simulink model "discret"  (R2020a)
settings: Solver=VariableStepAuto  StartTime=0.0  StopTime=0.03  RelTol=1e-3
undefined symbols (not defined in the file): K, Kfiltre, S, Te, Tg, Tr1, Tr2, Ubatt, Z0, Z00, Z1, Z11
settings Model: Creator=housni  LastModifiedBy=housni

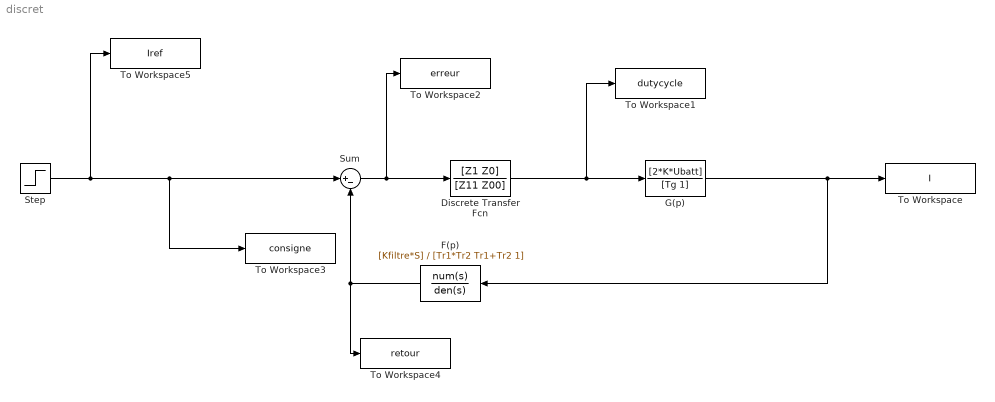
== system discret ==
  Discrete Transfer Fcn : DiscreteTransferFcn  Numerator=[Z1 Z0]  Denominator=[Z11 Z00]  SampleTime=Te
  F(p) : TransferFcn  Numerator=[Kfiltre*S]  Denominator=[Tr1*Tr2 Tr1+Tr2 1]
  G(p) : TransferFcn  Numerator=[2*K*Ubatt]  Denominator=[Tg 1]
  Step : Step  Time=0.01  SampleTime=0
  Sum : Sum  Inputs=|+-
  To Workspace : ToWorkspace  VariableName=I  SaveFormat=Timeseries  SampleTime=-1
  To Workspace1 : ToWorkspace  VariableName=dutycycle  SaveFormat=Timeseries  SampleTime=-1
  To Workspace2 : ToWorkspace  VariableName=erreur  SaveFormat=Timeseries  SampleTime=-1
  To Workspace3 : ToWorkspace  VariableName=consigne  SaveFormat=Timeseries  SampleTime=-1
  To Workspace4 : ToWorkspace  VariableName=retour  SaveFormat=Timeseries  SampleTime=-1
  To Workspace5 : ToWorkspace  VariableName=Iref  SaveFormat=Timeseries  SampleTime=-1
  wires:
  G(p)/1 -> F(p)/1, To Workspace/1
  F(p)/1 -> To Workspace4/1, Sum/2
  Step/1 -> To Workspace3/1, Sum/1, To Workspace5/1
  Sum/1 -> Discrete Transfer Fcn/1, To Workspace2/1
  Discrete Transfer Fcn/1 -> To Workspace1/1, G(p)/1
